simulink model "disc_model"  (R2023b)
settings: Solver=VariableStepAuto  StartTime=0.0  StopTime=15  RelTol=1e-3
undefined symbols (not defined in the file or in its folder): Ad, Bd, C, k1, k2, Kd, T, T2
settings Model: Creator=deniskirbaba  LastModifiedBy=deniskirbaba

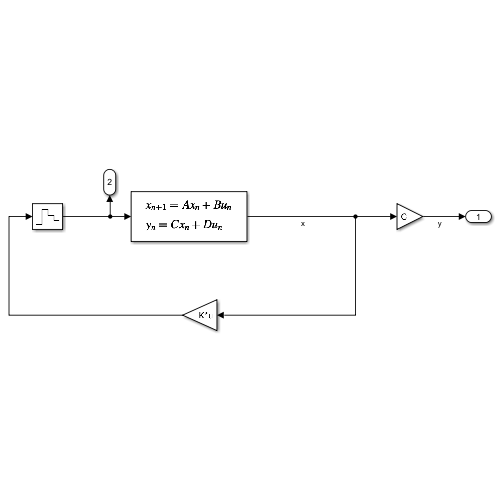
[thumbnail: Simulink's stored preview of the top-level diagram]
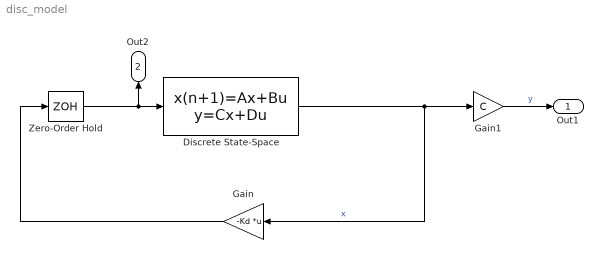
== system disc_model ==
  Discrete State-Space : DiscreteStateSpace  A=Ad  B=Bd  C=eye(2)  D=[0;0]  InitialCondition=[T2/k2*k1; 0]  SampleTime=-1
  Gain : Gain  Gain=-Kd  Multiplication=Matrix(K*u)
  Gain1 : Gain  Gain=C
  Zero-Order Hold : ZeroOrderHold  SampleTime=T
  Out1 : Outport
  Out2 : Outport  Port=2
  wires:
  Discrete State-Space/1 -> Gain1/1, Gain/1  "x"
  Gain/1 -> Zero-Order Hold/1
  Zero-Order Hold/1 -> Out2/1, Discrete State-Space/1
  Gain1/1 -> Out1/1  "y"
